simulink model "wahadlo_ultimate"  (R2016a)
settings: Solver=ode45  StartTime=0.0  StopTime=15  MaxStep=0.01  RelTol=1e-3
settings Model: Creator=ms36124  LastModifiedBy=ms36124

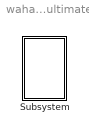
== system wahadlo_ultimate ==
  Subsystem : Subsystem  mask{g=9.81, k1=2, k2=1, m1=1, m2=2, l1=1, l2=2, f1=80, f2=150}

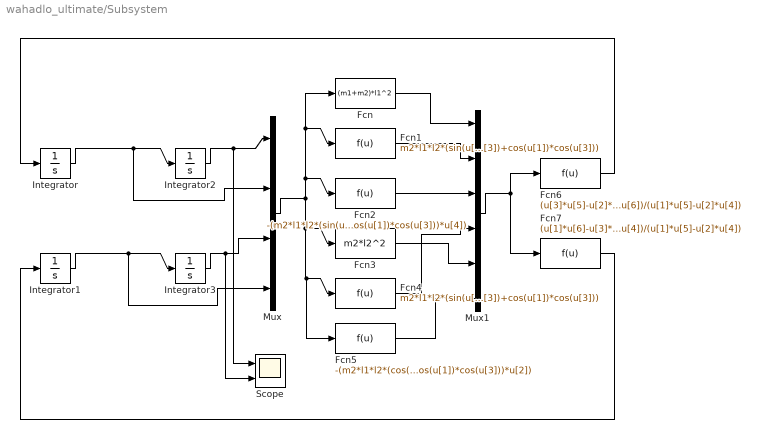
== system wahadlo_ultimate/Subsystem ==
  Fcn : Fcn  Expr=(m1+m2)*l1^2
  Fcn1 : Fcn  Expr=m2*l1*l2*(sin(u[1])*sin(u[3])+cos(u[1])*cos(u[3]))
  Fcn2 : Fcn  Expr=-(m2*l1*l2*(sin(u[1])*cos(u[3])-cos(u[1])*sin(u[3]))*u[4]^2+(m1+m2)*g*l1*sin(u[1])+k1*l1^2*u[2]+k2*l1*l2*(sin(u[1])*sin(u[3])+cos(u[1])*cos(u[3]))*u[4])
  Fcn3 : Fcn  Expr=m2*l2^2
  Fcn4 : Fcn  Expr=m2*l1*l2*(sin(u[1])*sin(u[3])+cos(u[1])*cos(u[3]))
  Fcn5 : Fcn  Expr=-(m2*l1*l2*(cos(u[1])*sin(u[3])-sin(u[1])*cos(u[3]))*u[2]^2+m2*g*l2*sin(u[3])+k2*l2^2*u[4]+k2*l1*l2*(sin(u[1])*sin(u[3])+cos(u[1])*cos(u[3]))*u[2])
  Fcn6 : Fcn  Expr=(u[3]*u[5]-u[2]*u[6])/(u[1]*u[5]-u[2]*u[4])
  Fcn7 : Fcn  Expr=(u[1]*u[6]-u[3]*u[4])/(u[1]*u[5]-u[2]*u[4])
  Integrator : Integrator
  Integrator1 : Integrator
  Integrator2 : Integrator  InitialCondition=f1*pi/180
  Integrator3 : Integrator  InitialCondition=f2*pi/180
  Mux : Mux
  Mux1 : Mux  Inputs=6
  Scope : Scope  NumInputPorts=2
  wires:
  Mux/1 -> Fcn2/1, Fcn1/1, Fcn/1, Fcn5/1, Fcn4/1, Fcn3/1
  Fcn/1 -> Mux1/1
  Fcn7/1 -> Integrator1/1
  Mux1/1 -> Fcn7/1, Fcn6/1
  Fcn3/1 -> Mux1/5
  Integrator3/1 -> Scope/2, Mux/3
  Integrator1/1 -> Mux/4, Integrator3/1
  Fcn4/1 -> Mux1/4
  Fcn2/1 -> Mux1/3
  Integrator2/1 -> Scope/1, Mux/1
  Fcn5/1 -> Mux1/6
  Integrator/1 -> Mux/2, Integrator2/1
  Fcn1/1 -> Mux1/2
  Fcn6/1 -> Integrator/1
